simulink model "MotorControl"  (R2017a)
settings: Solver=FixedStepDiscrete  StartTime=0.0  StopTime=1  FixedStep=0.001  RelTol=1e-3
values from neighbouring files (symbols this model uses):
  PWMValue = 1000.0    [MotorControl.sldd]
libraries: simulink x3
settings Model: DataDictionary=MotorControl.sldd  Creator=Administrator  LastModifiedBy=Administrator
settings OptimizationCC: DefaultParameterBehavior=Inlined  PassReuseOutputArgsAs=Individual arguments
settings DebuggingCC: ParameterTunabilityLossMsg=error
settings SFSimCC: MATLABDynamicMemAlloc=off
settings RTWCC: SystemTargetFile=ert.tlc  GenCodeOnly=on  TemplateMakefile=ert_default_tmf  Description=Embedded Coder  GenerateReport=on  IncludeHyperlinkInReport=on  LaunchReport=on  GenerateTraceInfo=on  GenerateTraceReport=on  GenerateTraceReportSl=on  GenerateTraceReportSf=on  GenerateTraceReportEml=on
settings CodeAppCC: ForceParamTrailComments=on  IgnoreCustomStorageClasses=off  OperatorAnnotations=on  SimulinkDataObjDesc=on  SFDataObjDesc=on  MATLABFcnDesc=on  InsertBlockDesc=on  MATLABSourceComments=on
settings ERTTargetCC: TargetLangStandard=C99 (ISO)  InlinedParameterPlacement=NonHierarchical  ERTCustomFileTemplate=example_file_process.tlc

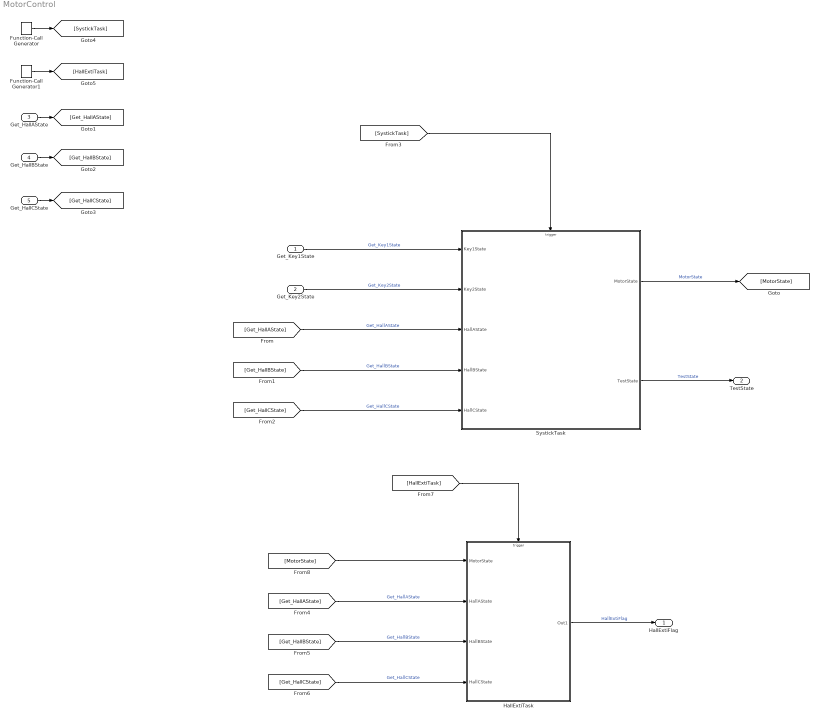
== system MotorControl ==
  Get_Key1State : Inport
  Get_Key2State : Inport  Port=2
  Get_HallAState : Inport  Port=3
  Get_HallBState : Inport  Port=4
  Get_HallCState : Inport  Port=5
  Function-Call Generator : simulink/Ports & Subsystems/Function-Call Generator  sample_time=0.001  numberOfIterations=1
  Function-Call Generator1 : simulink/Ports & Subsystems/Function-Call Generator  sample_time=-1  numberOfIterations=1
  HallExtiTask : Subsystem  TreatAsAtomicUnit=on  RTWFcnName=HallExtiTask  RTWFileName=HallExtiTask
      settings: RTWSystemCode=Nonreusable function  RTWFcnNameOpts=User specified  RTWFileNameOpts=User specified
  SystickTask : Subsystem  TreatAsAtomicUnit=on  RTWFcnName=SystickTask  RTWFileName=SystickTask
      settings: RTWSystemCode=Nonreusable function  RTWFcnNameOpts=User specified  RTWFileNameOpts=User specified
  HallExtiFlag : Outport
  TestState : Outport  Port=2
  wires:
  SystickTask/1(MotorState) -> [MotorState]  "MotorState"
  HallExtiTask/1(Out1) -> HallExtiFlag/1  "HallExtiFlag"
  [SystickTask] -> SystickTask/Trigger
  [Get_HallAState] -> SystickTask/3(HallAState)  "Get_HallAState"
  [Get_HallCState] -> SystickTask/5(HallCState)  "Get_HallCState"
  [Get_HallBState] -> SystickTask/4(HallBState)  "Get_HallBState"
  Get_Key2State/1 -> SystickTask/2(Key2State)  "Get_Key2State"
  Get_Key1State/1 -> SystickTask/1(Key1State)  "Get_Key1State"
  [HallExtiTask] -> HallExtiTask/Trigger
  [Get_HallCState] -> HallExtiTask/4(HallCState)  "Get_HallCState"
  [Get_HallBState] -> HallExtiTask/3(HallBState)  "Get_HallBState"
  [Get_HallAState] -> HallExtiTask/2(HallAState)  "Get_HallAState"
  [MotorState] -> HallExtiTask/1(MotorState)
  Get_HallAState/1 -> [Get_HallAState]
  Get_HallBState/1 -> [Get_HallBState]
  Get_HallCState/1 -> [Get_HallCState]
  Function-Call Generator/1 -> [SystickTask]
  Function-Call Generator1/1 -> [HallExtiTask]
  SystickTask/2(TestState) -> TestState/1  "TestState"

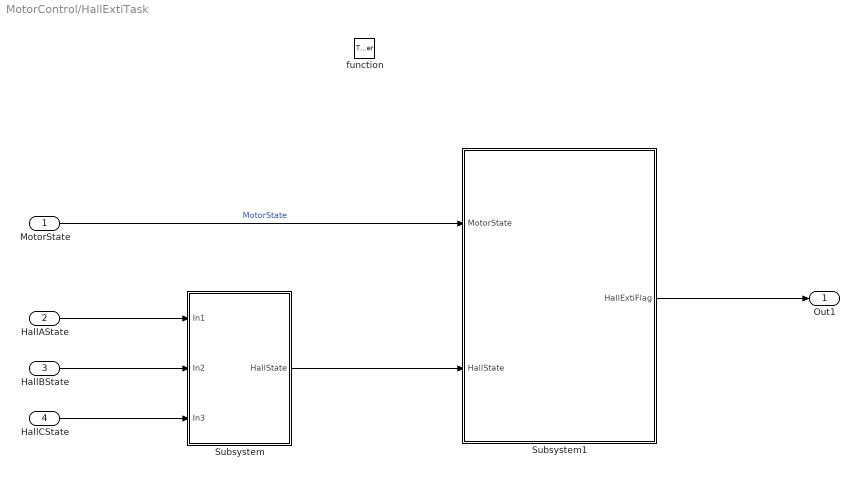
== system MotorControl/HallExtiTask ==
  MotorState : Inport
  HallAState : Inport  Port=2
  HallBState : Inport  Port=3
  HallCState : Inport  Port=4
  function : TriggerPort  TriggerType=function-call  VariantControl=Variant
  Subsystem : Subsystem
  Subsystem1 : Subsystem
  Out1 : Outport
  wires:
  HallBState/1 -> Subsystem/2(In2)
  HallAState/1 -> Subsystem/1(In1)
  HallCState/1 -> Subsystem/3(In3)
  MotorState/1 -> Subsystem1/1(MotorState)  "MotorState"
  Subsystem/1(HallState) -> Subsystem1/2(HallState)
  Subsystem1/1(HallExtiFlag) -> Out1/1

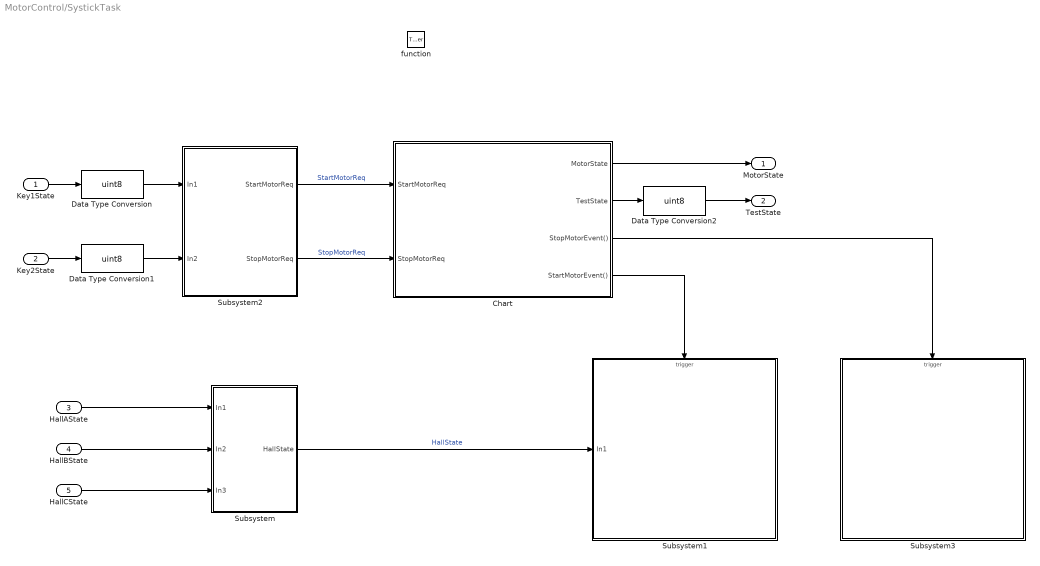
== system MotorControl/SystickTask ==
  Key1State : Inport
  Key2State : Inport  Port=2
  HallAState : Inport  Port=3
  HallBState : Inport  Port=4
  HallCState : Inport  Port=5
  function : TriggerPort  TriggerType=function-call  VariantControl=Variant
  Chart : Stateflow chart  TreatAsAtomicUnit=on
  Data Type Conversion : DataTypeConversion  OutDataTypeStr=uint8
  Data Type Conversion1 : DataTypeConversion  OutDataTypeStr=uint8
  Data Type Conversion2 : DataTypeConversion  OutDataTypeStr=uint8
  Subsystem : Subsystem
  Subsystem1 : Subsystem
  Subsystem2 : Subsystem
  Subsystem3 : Subsystem
  MotorState : Outport
  TestState : Outport  Port=2
  wires:
  Key1State/1 -> Data Type Conversion/1
  Key2State/1 -> Data Type Conversion1/1
  Subsystem2/1(StartMotorReq) -> Chart/1(StartMotorReq)  "StartMotorReq"
  Subsystem2/2(StopMotorReq) -> Chart/2(StopMotorReq)  "StopMotorReq"
  Chart/1(MotorState) -> MotorState/1
  HallAState/1 -> Subsystem/1(In1)
  HallBState/1 -> Subsystem/2(In2)
  HallCState/1 -> Subsystem/3(In3)
  Subsystem/1(HallState) -> Subsystem1/1(In1)  "HallState"
  Chart/4(StartMotorEvent()) -> Subsystem1/Trigger
  Chart/3(StopMotorEvent()) -> Subsystem3/Trigger
  Data Type Conversion/1 -> Subsystem2/1(In1)
  Data Type Conversion1/1 -> Subsystem2/2(In2)
  Chart/2(TestState) -> Data Type Conversion2/1
  Data Type Conversion2/1 -> TestState/1

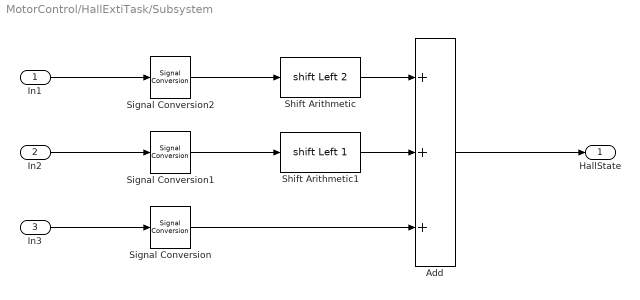
== system MotorControl/HallExtiTask/Subsystem ==
  In1 : Inport
  In2 : Inport  Port=2
  In3 : Inport  Port=3
  Add : Sum  Inputs=+++
  Shift Arithmetic : ArithShift  BitShiftNumber=2  BitShiftDirection=Left
  Shift Arithmetic1 : ArithShift  BitShiftNumber=1  BitShiftDirection=Left
  Signal Conversion : SignalConversion  OverrideOpt=off
  Signal Conversion1 : SignalConversion  OverrideOpt=off
  Signal Conversion2 : SignalConversion  OverrideOpt=on
  HallState : Outport
  wires:
  Add/1 -> HallState/1
  Signal Conversion/1 -> Add/3
  In3/1 -> Signal Conversion/1
  Signal Conversion1/1 -> Shift Arithmetic1/1
  Signal Conversion2/1 -> Shift Arithmetic/1
  Shift Arithmetic/1 -> Add/1
  In1/1 -> Signal Conversion2/1
  In2/1 -> Signal Conversion1/1
  Shift Arithmetic1/1 -> Add/2

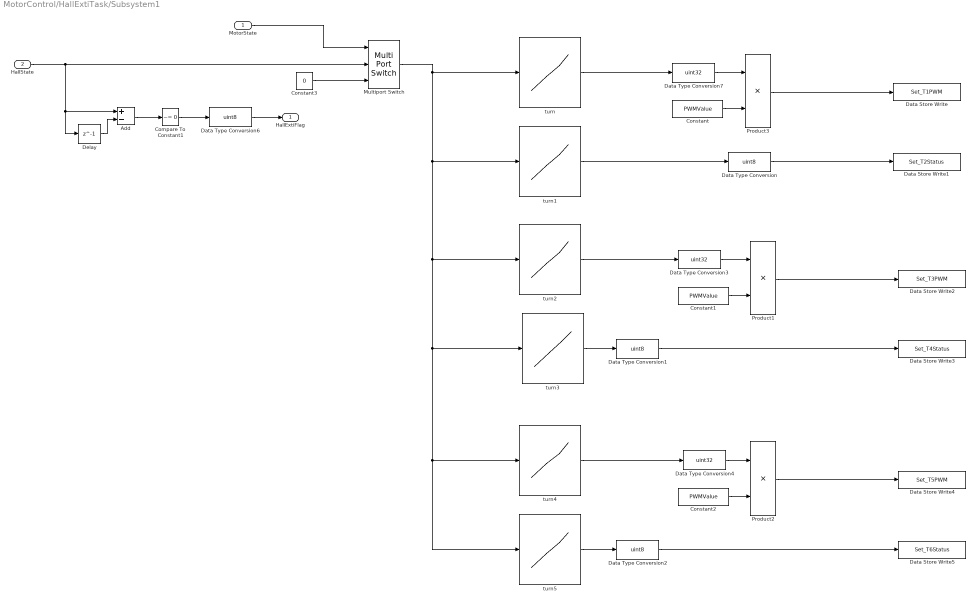
== system MotorControl/HallExtiTask/Subsystem1 ==
  MotorState : Inport
  HallState : Inport  Port=2
  Add : Sum  Inputs=+-
  Compare To Constant1 : simulink/Logic and Bit Operations/Compare To Constant  relop=~=  const=0  OutDataTypeStr=boolean
  Constant : Constant  Value=PWMValue
  Constant1 : Constant  Value=PWMValue
  Constant2 : Constant  Value=PWMValue
  Constant3 : Constant  Value=0  OutDataTypeStr=uint8
  Data Store Write : DataStoreWrite  DataStoreName=Set_T1PWM
  Data Store Write1 : DataStoreWrite  DataStoreName=Set_T2Status
  Data Store Write2 : DataStoreWrite  DataStoreName=Set_T3PWM
  Data Store Write3 : DataStoreWrite  DataStoreName=Set_T4Status
  Data Store Write4 : DataStoreWrite  DataStoreName=Set_T5PWM
  Data Store Write5 : DataStoreWrite  DataStoreName=Set_T6Status
  Data Type Conversion{,1..2,6} (4 alike) : DataTypeConversion  OutDataTypeStr=uint8
  Data Type Conversion3 : DataTypeConversion  OutDataTypeStr=uint32
  Data Type Conversion4 : DataTypeConversion  OutDataTypeStr=uint32
  Data Type Conversion7 : DataTypeConversion  OutDataTypeStr=uint32
  Delay : Delay  DelayLength=1  InitialCondition=0
  Multiport Switch : MultiPortSwitch  DataPortOrder=Specify indices  DataPortIndices={Enum_MotorState.Run,Enum_MotorState.Init}
  Product1 : Product  OutDataTypeStr=uint32
  Product2 : Product  OutDataTypeStr=uint32
  Product3 : Product  OutDataTypeStr=uint32
  turn : Lookup_n-D  NumberOfTableDimensions=1  BreakpointsForDimension1=[0 1 2 3 4 5 6]  Table=[0 0 0 0 1 1 0]  InterpMethod=Nearest  InternalRulePriority=Speed  RndMeth=Simplest  InputSameDT=on
  turn1 : Lookup_n-D  NumberOfTableDimensions=1  BreakpointsForDimension1=[0 1 2 3 4 5 6]  Table=[0 0 1 1 0 0 0 ]  InterpMethod=Nearest  InternalRulePriority=Speed  RndMeth=Simplest  InputSameDT=on
  turn2 : Lookup_n-D  NumberOfTableDimensions=1  BreakpointsForDimension1=[0 1 2 3 4 5 6]  Table=[0 0 1 0 0 0 1]  InterpMethod=Nearest  InternalRulePriority=Speed  RndMeth=Simplest  InputSameDT=on
  turn3 : Lookup_n-D  NumberOfTableDimensions=1  BreakpointsForDimension1=[0 1 2 3 4 5 6]  Table=[0 1 0 0 0 1 0]  InterpMethod=Nearest  InternalRulePriority=Speed  RndMeth=Simplest  InputSameDT=on
  turn4 : Lookup_n-D  NumberOfTableDimensions=1  BreakpointsForDimension1=[0 1 2 3 4 5 6]  Table=[0 1 0 1 0 0 0]  InterpMethod=Nearest  InternalRulePriority=Speed  RndMeth=Simplest  InputSameDT=on
  turn5 : Lookup_n-D  NumberOfTableDimensions=1  BreakpointsForDimension1=[0 1 2 3 4 5 6]  Table=[0 0 0 0 1 0 1]  InterpMethod=Nearest  InternalRulePriority=Speed  RndMeth=Simplest  InputSameDT=on
  HallExtiFlag : Outport
  wires:
  Constant2/1 -> Product2/2
  turn5/1 -> Data Type Conversion2/1
  Product2/1 -> Data Store Write4/1
  Data Type Conversion2/1 -> Data Store Write5/1
  turn4/1 -> Data Type Conversion4/1
  turn1/1 -> Data Type Conversion/1
  Multiport Switch/1 -> turn4/1, turn5/1, turn3/1, turn2/1, turn1/1, turn/1
  Data Type Conversion/1 -> Data Store Write1/1
  turn3/1 -> Data Type Conversion1/1
  Constant1/1 -> Product1/2
  turn2/1 -> Data Type Conversion3/1
  Product1/1 -> Data Store Write2/1
  Data Type Conversion1/1 -> Data Store Write3/1
  Product3/1 -> Data Store Write/1
  turn/1 -> Data Type Conversion7/1
  Constant/1 -> Product3/2
  Delay/1 -> Add/2
  Add/1 -> Compare To Constant1/1
  MotorState/1 -> Multiport Switch/1
  HallState/1 -> Multiport Switch/2, Add/1, Delay/1
  Compare To Constant1/1 -> Data Type Conversion6/1
  Data Type Conversion6/1 -> HallExtiFlag/1
  Data Type Conversion7/1 -> Product3/1
  Data Type Conversion3/1 -> Product1/1
  Data Type Conversion4/1 -> Product2/1
  Constant3/1 -> Multiport Switch/3

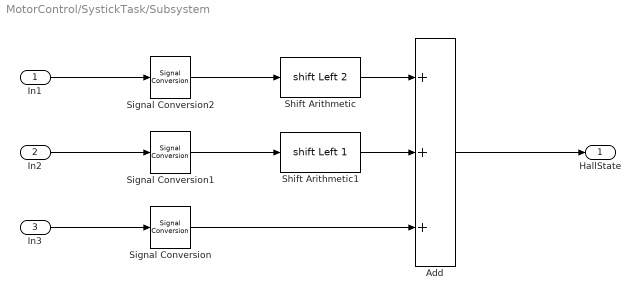
== system MotorControl/SystickTask/Subsystem ==
  In1 : Inport
  In2 : Inport  Port=2
  In3 : Inport  Port=3
  Add : Sum  Inputs=+++
  Shift Arithmetic : ArithShift  BitShiftNumber=2  BitShiftDirection=Left
  Shift Arithmetic1 : ArithShift  BitShiftNumber=1  BitShiftDirection=Left
  Signal Conversion : SignalConversion  OverrideOpt=off
  Signal Conversion1 : SignalConversion  OverrideOpt=off
  Signal Conversion2 : SignalConversion  OverrideOpt=off
  HallState : Outport
  wires:
  Add/1 -> HallState/1
  Signal Conversion/1 -> Add/3
  In3/1 -> Signal Conversion/1
  Signal Conversion1/1 -> Shift Arithmetic1/1
  Signal Conversion2/1 -> Shift Arithmetic/1
  Shift Arithmetic/1 -> Add/1
  In1/1 -> Signal Conversion2/1
  In2/1 -> Signal Conversion1/1
  Shift Arithmetic1/1 -> Add/2

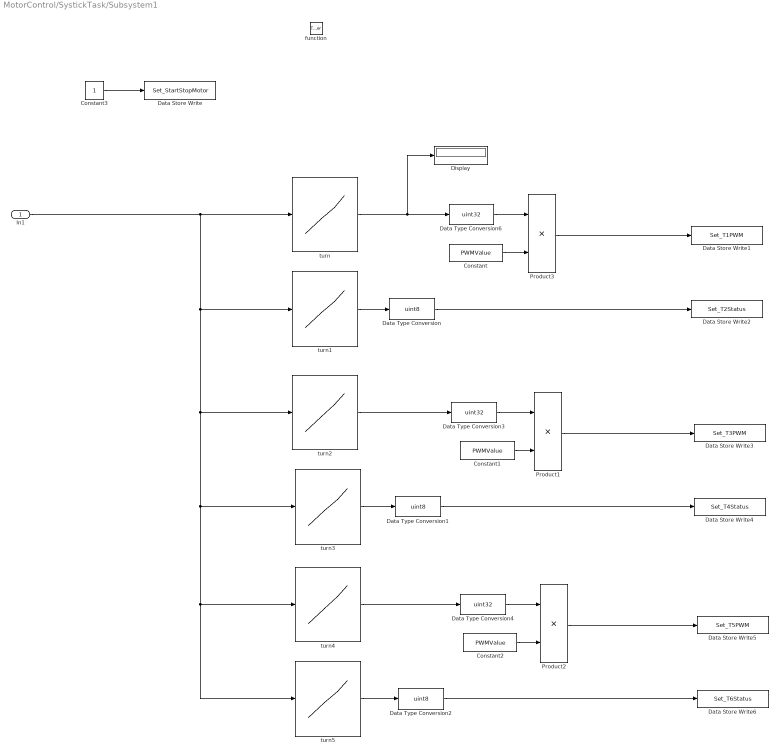
== system MotorControl/SystickTask/Subsystem1 ==
  In1 : Inport
  function : TriggerPort  TriggerType=function-call  VariantControl=Variant
  Constant : Constant  Value=PWMValue
  Constant1 : Constant  Value=PWMValue
  Constant2 : Constant  Value=PWMValue
  Constant3 : Constant  OutDataTypeStr=uint8
  Data Store Write : DataStoreWrite  Priority=0  DataStoreName=Set_StartStopMotor
  Data Store Write1 : DataStoreWrite  DataStoreName=Set_T1PWM
  Data Store Write2 : DataStoreWrite  DataStoreName=Set_T2Status
  Data Store Write3 : DataStoreWrite  DataStoreName=Set_T3PWM
  Data Store Write4 : DataStoreWrite  DataStoreName=Set_T4Status
  Data Store Write5 : DataStoreWrite  DataStoreName=Set_T5PWM
  Data Store Write6 : DataStoreWrite  DataStoreName=Set_T6Status
  Data Type Conversion : DataTypeConversion  OutDataTypeStr=uint8
  Data Type Conversion1 : DataTypeConversion  OutDataTypeStr=uint8
  Data Type Conversion2 : DataTypeConversion  OutDataTypeStr=uint8
  Data Type Conversion3 : DataTypeConversion  OutDataTypeStr=uint32
  Data Type Conversion4 : DataTypeConversion  OutDataTypeStr=uint32
  Data Type Conversion6 : DataTypeConversion  OutDataTypeStr=uint32
  Display : Display
  Product1 : Product  OutDataTypeStr=uint32
  Product2 : Product  OutDataTypeStr=uint32
  Product3 : Product  OutDataTypeStr=uint32
  turn : Lookup_n-D  NumberOfTableDimensions=1  BreakpointsForDimension1=[1 2 3 4 5 6]  Table=[0 0 0 1 1 0]  InterpMethod=Nearest  InternalRulePriority=Speed  RndMeth=Simplest  InputSameDT=on
  turn1 : Lookup_n-D  NumberOfTableDimensions=1  BreakpointsForDimension1=[1 2 3 4 5 6]  Table=[0 1 1 0 0 0 ]  InterpMethod=Nearest  InternalRulePriority=Speed  RndMeth=Simplest  InputSameDT=on
  turn2 : Lookup_n-D  NumberOfTableDimensions=1  BreakpointsForDimension1=[1 2 3 4 5 6]  Table=[0 1 0 0 0 1]  InterpMethod=Nearest  InternalRulePriority=Speed  RndMeth=Simplest  InputSameDT=on
  turn3 : Lookup_n-D  NumberOfTableDimensions=1  BreakpointsForDimension1=[1 2 3 4 5 6]  Table=[1 0 0 0 1 0]  InterpMethod=Nearest  InternalRulePriority=Speed  RndMeth=Simplest  InputSameDT=on
  turn4 : Lookup_n-D  NumberOfTableDimensions=1  BreakpointsForDimension1=[1 2 3 4 5 6]  Table=[1 0 1 0 0 0]  InterpMethod=Nearest  InternalRulePriority=Speed  RndMeth=Simplest  InputSameDT=on
  turn5 : Lookup_n-D  NumberOfTableDimensions=1  BreakpointsForDimension1=[1 2 3 4 5 6]  Table=[0 0 0 1 0 1]  InterpMethod=Nearest  InternalRulePriority=Speed  RndMeth=Simplest  InputSameDT=on
  wires:
  Constant3/1 -> Data Store Write/1
  Product2/1 -> Data Store Write5/1
  Constant1/1 -> Product1/2
  Data Type Conversion2/1 -> Data Store Write6/1
  turn3/1 -> Data Type Conversion1/1
  turn5/1 -> Data Type Conversion2/1
  Constant2/1 -> Product2/2
  Constant/1 -> Product3/2
  Data Type Conversion6/1 -> Product3/1
  Data Type Conversion1/1 -> Data Store Write4/1
  Product3/1 -> Data Store Write1/1
  In1/1 -> turn1/1, turn3/1, turn4/1, turn5/1, turn2/1, turn/1
  Data Type Conversion/1 -> Data Store Write2/1
  turn1/1 -> Data Type Conversion/1
  turn2/1 -> Data Type Conversion3/1
  Data Type Conversion3/1 -> Product1/1
  Data Type Conversion4/1 -> Product2/1
  turn4/1 -> Data Type Conversion4/1
  turn/1 -> Display/1, Data Type Conversion6/1
  Product1/1 -> Data Store Write3/1

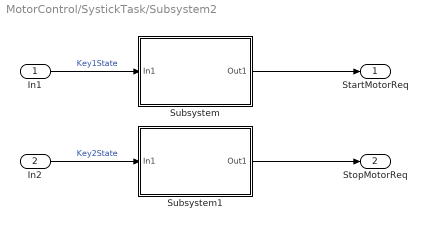
== system MotorControl/SystickTask/Subsystem2 ==
  In1 : Inport
  In2 : Inport  Port=2
  Subsystem : Subsystem
  Subsystem1 : Subsystem
  StartMotorReq : Outport
  StopMotorReq : Outport  Port=2
  wires:
  Subsystem/1(Out1) -> StartMotorReq/1
  Subsystem1/1(Out1) -> StopMotorReq/1
  In2/1 -> Subsystem1/1(In1)  "Key2State"
  In1/1 -> Subsystem/1(In1)  "Key1State"

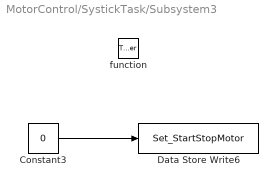
== system MotorControl/SystickTask/Subsystem3 ==
  function : TriggerPort  TriggerType=function-call  VariantControl=Variant
  Constant3 : Constant  Value=0  OutDataTypeStr=uint8
  Data Store Write6 : DataStoreWrite  DataStoreName=Set_StartStopMotor
  wires:
  Constant3/1 -> Data Store Write6/1

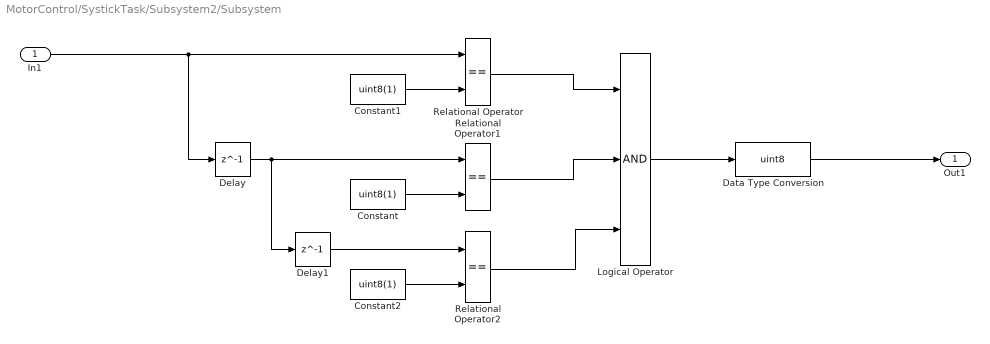
== system MotorControl/SystickTask/Subsystem2/Subsystem ==
  In1 : Inport
  Constant : Constant  Value=uint8(1)
  Constant1 : Constant  Value=uint8(1)
  Constant2 : Constant  Value=uint8(1)
  Data Type Conversion : DataTypeConversion  OutDataTypeStr=uint8
  Delay : Delay  DelayLength=1  InitialCondition=0
  Delay1 : Delay  DelayLength=1  InitialCondition=0
  Logical Operator : Logic  Inputs=3  AllPortsSameDT=off  OutDataTypeStr=boolean
  Relational Operator : RelationalOperator  Operator===  OutDataTypeStr=boolean  RndMeth=Simplest
  Relational Operator1 : RelationalOperator  Operator===  OutDataTypeStr=boolean  RndMeth=Simplest
  Relational Operator2 : RelationalOperator  Operator===  OutDataTypeStr=boolean  RndMeth=Simplest
  Out1 : Outport
  wires:
  Constant2/1 -> Relational Operator2/2
  Delay/1 -> Delay1/1, Relational Operator1/1
  Constant1/1 -> Relational Operator/2
  Relational Operator2/1 -> Logical Operator/3
  Relational Operator1/1 -> Logical Operator/2
  Relational Operator/1 -> Logical Operator/1
  Constant/1 -> Relational Operator1/2
  In1/1 -> Delay/1, Relational Operator/1
  Delay1/1 -> Relational Operator2/1
  Logical Operator/1 -> Data Type Conversion/1
  Data Type Conversion/1 -> Out1/1

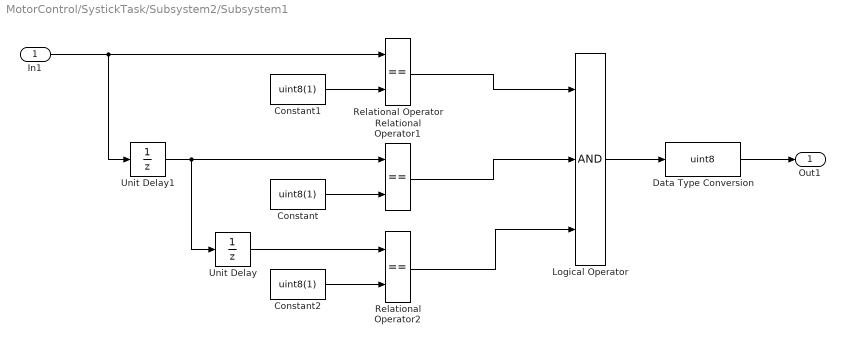
== system MotorControl/SystickTask/Subsystem2/Subsystem1 ==
  In1 : Inport
  Constant : Constant  Value=uint8(1)
  Constant1 : Constant  Value=uint8(1)
  Constant2 : Constant  Value=uint8(1)
  Data Type Conversion : DataTypeConversion  OutDataTypeStr=uint8
  Logical Operator : Logic  Inputs=3  AllPortsSameDT=off  OutDataTypeStr=boolean
  Relational Operator : RelationalOperator  Operator===  OutDataTypeStr=boolean  RndMeth=Simplest
  Relational Operator1 : RelationalOperator  Operator===  OutDataTypeStr=boolean  RndMeth=Simplest
  Relational Operator2 : RelationalOperator  Operator===  OutDataTypeStr=boolean  RndMeth=Simplest
  Unit Delay : UnitDelay  SampleTime=-1
  Unit Delay1 : UnitDelay  SampleTime=-1
  Out1 : Outport
  wires:
  Data Type Conversion/1 -> Out1/1
  Logical Operator/1 -> Data Type Conversion/1
  Unit Delay/1 -> Relational Operator2/1
  In1/1 -> Relational Operator/1, Unit Delay1/1
  Constant/1 -> Relational Operator1/2
  Relational Operator/1 -> Logical Operator/1
  Relational Operator1/1 -> Logical Operator/2
  Relational Operator2/1 -> Logical Operator/3
  Constant1/1 -> Relational Operator/2
  Unit Delay1/1 -> Relational Operator1/1, Unit Delay/1
  Constant2/1 -> Relational Operator2/2

== stateflow chart MotorControl/SystickTask/Chart ==
  state Init
    en:
    MotorState = Enum_MotorState.Init;
    TestState = 1;
  state Start
    en:
    MotorState = Enum_MotorState.Start;
    StartCount = 0;
    StartMotorEvent;
    TestState = 2;
    du:
    StartCount = StartCount + 1;
  state Stop
    en:
    MotorState = Enum_MotorState.Stop;
    StopMotorEvent;
    TestState = 4;
  state Run
    en:
    MotorState = Enum_MotorState.Run;
    StartCount = 0;
    TestState = 3;
  (default) -> Init
  Init -> Start : [StartMotorReq == 1]
  Stop -> Start : [StartMotorReq == 1]
  Start -> Stop [order 2] : [StopMotorReq == 1]
  Start -> Run [order 1] : [StartCount == 10]
  Run -> Stop : [StopMotorReq == 1]
  data: StartMotorReq input; StopMotorReq input; MotorState output; StartCount local; TestState output
  events: StopMotorEvent output FUNCTION_CALL_EVENT; StartMotorEvent output FUNCTION_CALL_EVENT
